simulink model "house_without_controller_sim"  (R2020b)
settings: Solver=ode45  StartTime=0.0  StopTime=4*3600  RelTol=1e-3  EnableMultiTasking=on
undefined symbols (not defined in the file): C_R, K, Q_F_ON, Q_H, t_a, t_init, tau_F
settings Model: Creator=sgt  LastModifiedBy=Hammer
settings DataIOCC: LimitDataPoints=on  SaveFormat=Array  SignalLoggingSaveFormat=ModelDataLogs
settings OptimizationCC: ExpressionDepthLimit=2147483647  InitFltsAndDblsToZero=on  LifeSpan=inf
settings DebuggingCC: SaveWithParameterizedLinksMsg=none  UnderspecifiedInitializationDetection=Classic  MergeDetectMultiDrivingBlocksExec=none  SignalResolutionControl=TryResolveAllWithWarning  SolverPrmCheckMsg=warning  MultiTaskDSMMsg=warning  MultiTaskCondExecSysMsg=none  StateNameClashWarn=warning  SFUnexpectedBacktrackingDiag=warning  SFNoUnconditionalDefaultTransitionDiag=warning  SFExecutionAtInitializationDiag=none  ArithmeticOperatorsInVariantConditions=warning
settings HardwareCC: ProdBitPerPointer=32  ProdBitPerSizeT=32  ProdBitPerPtrDiffT=32  ProdLargestAtomicFloat=None  ProdIntDivRoundTo=Undefined  ProdEndianess=Unspecified  ProdWordSize=32  ProdHWDeviceType=32-bit Generic
settings ModelReferenceCC: PropagateSignalLabelsOutOfModel=off
settings SFSimCC: SimUseLocalCustomCode=off  CustomCodeUndefinedFunction=UseInterfaceOnly
settings RTWCC: RTWUseLocalCustomCode=off
settings CodeAppCC: StateflowObjectComments=on
settings GRTTargetCC: TargetFcnLib=ansi_tfl_tmw.mat  TargetLangStandard=C89/C90 (ANSI)  CombineOutputUpdateFcns=off  GRTInterface=on
settings ConfigComp: CovMetricSettings=dw  CovSaveCumulativeToWorkspaceVar=on  CovSaveSingleToWorkspaceVar=on  CovExternalEMLEnable=off

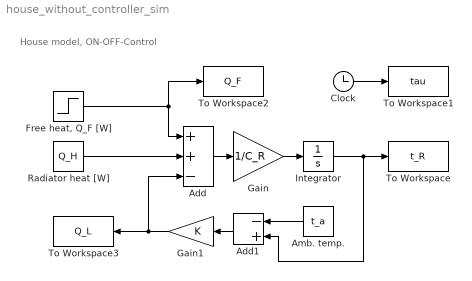
== system house_without_controller_sim ==
  note: House model, ON-OFF-Control
  Add : Sum  Inputs=++-
  Add1 : Sum  Inputs=-+
  Amb. temp. : Constant  Value=t_a
  Clock : Clock
  "Free heat, Q_F [W]" : Step  Time=tau_F  After=Q_F_ON  SampleTime=0
  Gain : Gain  Gain=1/C_R
  Gain1 : Gain  Gain=K
  Integrator : Integrator  InitialCondition=t_init
  Radiator heat [W] : Constant  Value=Q_H
  To Workspace : ToWorkspace  VariableName=t_R  SampleTime=-1
  To Workspace1 : ToWorkspace  VariableName=tau  SampleTime=-1
  To Workspace2 : ToWorkspace  VariableName=Q_F  SampleTime=-1
  To Workspace3 : ToWorkspace  VariableName=Q_L  SampleTime=-1
  wires:
  Integrator/1 -> Add1/2, To Workspace/1
  Clock/1 -> To Workspace1/1
  Gain/1 -> Integrator/1
  Add/1 -> Gain/1
  "Free heat, Q_F [W]"/1 -> Add/1, To Workspace2/1
  Amb. temp./1 -> Add1/1
  Add1/1 -> Gain1/1
  Gain1/1 -> Add/3, To Workspace3/1
  Radiator heat [W]/1 -> Add/2
